simulink model "proje_v1"  (R2016a)
settings: Solver=VariableStepAuto  StartTime=0.0  StopTime=2  RelTol=1e-3
libraries: powerlib x7, electricdrivelib x1
settings Model: Creator=acer  LastModifiedBy=gunge

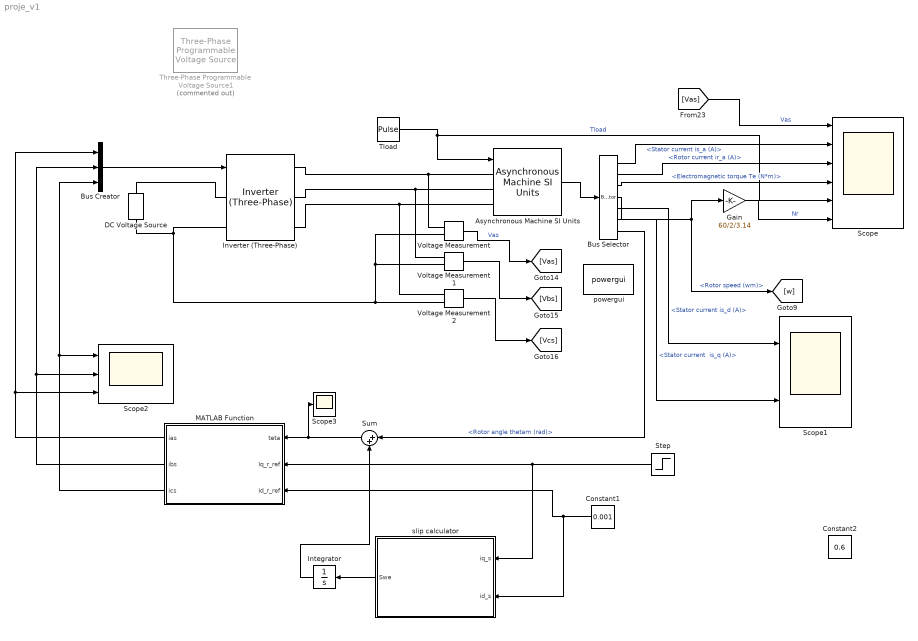
== system proje_v1 ==
  Asynchronous Machine SI Units : powerlib/Machines/Asynchronous Machine SI Units  RotorType=Squirrel-cage  PresetModel=No  MechanicalLoad=Torque Tm  ShowDetailedParameters=on  ReferenceFrame=Rotor  Units=SI  MeasurementBus=off  NominalParameters=[3730 230 60]  Stator=[0.531 0.00252]  Rotor=[0.408 0.00252]  Cage1=[0.4155 0.002066]  Cage2=[0.4168 0.0003495]  Lm=0.0847  Mechanical=[0.1 0 2]  PolePairs=2  InitialConditions=[1 0 0 0 0 0 0 0]  SimulateSaturation=off  Saturation=[14.03593122, 27.81365428, 53.79336849, 72.68890987, 97.98006896, 148.6815601, 215.7428561, 302.9841135, 428.7778367 ; 230, 322, 414, 460, 506, 552, 598, 644, 690]  LoadFlowParameters=1492000  TsPowergui=0  TsBlock=-1  IterativeModel=Trapezoidal non iterative  IterativeDiscreteModel=Trapezoidal non iterative  Pmec=1.492e+006
  Bus Creator : BusCreator  Inputs=3
  Bus Selector : BusSelector  OutputSignals="Stator measurements.Stator current is_a (A),Rotor measurements.Rotor current ir_a (A),Mechanical.Electromagnetic torque Te (N*m),Mechanical.Rotor speed (wm),Stator measurements.Stator current is_d (A),Stator measurements.Stator current  is_q (A),Mechanical.Rotor angle thetam (rad)"
  Constant1 : Constant  Value=0.001
  Constant2 : Constant  Value=0.6
  DC Voltage Source : powerlib/Electrical Sources/DC Voltage Source  Amplitude=540  Measurements=Voltage
  Gain : Gain  Gain=60/2/3.14
  Integrator : Integrator
  Inverter (Three-Phase) : electricdrivelib/Fundamental Drive Blocks/Inverter (Three-Phase)  OverrideUsingVariant=Average_SVM  detailLevel=Average  driveType=Space vector modulation  Ts=2e-6  SnubberResistance=10e3  SnubberCapacitance=inf  Device=IGBT / Diodes  Ron=1e-3  ForwardVoltages=[1.2,1.2]  GTOparameters=[1e-6,2e-6]  IGBTparameters=[1e-6,2e-6]  Measurements=All voltages and currents  converterType=Inverter  SourceFrequency=60  ReferenceFrame=Rotor  dqInductances=[8.5e-3,8.5e-3]  Inductance=8.5e-3  Ls=0  Resistance=0.2  Flux=0.175  Stator_sm=[2.01e-3,4.289e-4,4.477e-3,1.354e-3]  Stator_im=[14.85e-3,0.3027e-3]  Rotor=[9.295e-3,0.3027e-3]  Lm=10.46e-3  p=4
      settings: AttributesFormatString=%<BlockChoice>
  MATLAB Function : MATLAB Function  TreatAsAtomicUnit=on
  Scope : Scope  NumInputPorts=6
  Scope1 : Scope  NumInputPorts=2
  Scope2 : Scope  NumInputPorts=3
  Scope3 : Scope
  Step : Step  Before=0.3  After=0.6  SampleTime=0
  Sum : Sum  Inputs=|++
  Three-Phase Programmable Voltage Source1 : powerlib/Electrical Sources/Three-Phase Programmable Voltage Source  Commented=on  PositiveSequence="[230  0 60]"  VariationEntity=None  VariationType=Table of time-amplitude pairs  VariationTypeAlt=Step  VariationStep=0.5  VariationRate=10  VariationMagnitude=0.3  VariationFrequency=2  VariationTiming=[1 2]  VariationPhaseA=off  Amplitudes=[1 0.8 1.2 1.0]  TimeValues=[0 0.1 0.15 0.2]  HarmonicGeneration=off  HarmonicA=[3 0.2 -25 0]  HarmonicB=[2 0.15 35 2]  Timing="[0.05  3]"  BusType=swing  Pref=0  Qref=0  Qmin=-inf  Qmax=inf
  Tload : DiscretePulseGenerator  PulseType=Time based  Amplitude=15  Period=1  PulseWidth=10  PhaseDelay=0.7
  Voltage Measurement : powerlib/Measurements/Voltage Measurement  PhasorSimulation=off  OutputType=Complex  PSBequivalent=0
  Voltage Measurement1 : powerlib/Measurements/Voltage Measurement  PhasorSimulation=off  OutputType=Complex  PSBequivalent=0
  Voltage Measurement2 : powerlib/Measurements/Voltage Measurement  PhasorSimulation=off  OutputType=Complex  PSBequivalent=0
  powergui : powerlib/powergui  Priority=1  SimulationMode=Discrete  SolverType=Tustin/Backward Euler (TBE)  SampleTime=1e-6  frequency=60  SPID=off  DisableSnubberDevices=off  DisableRonSwitches=off  DisableVfSwitches=off  SwTol=0  DisplayEquations=off  Interpol=off  ExternalGateDelay=off  methode=off  Ts=10  FunctionMessages=off  echomessages=off  HookPort=off  EnableUseOfTLC=off  x0status=blocks  frequencyindice=60  Pbase=100e6  ErrMax=1e-4  Iterations=50  UnitsV=kV  UnitsW=MW  buscounter=0  RestoreLinks=warning  ResistiveCurrentMeasurement=off  Frange=[0:2:500]  Ylog=off  Xlog=on  ShowGrid=off  save=off  variable=ZData  structure=0  ZoomFFT=off  StartTime=0.0  cycles=1  DisplayStyle=1  fundamental=60  FreqAxis=off  MaxFrequency=1000  frequencyindicesteady=1  RmsSteady=1  display=off
  slip calculator : MATLAB Function  TreatAsAtomicUnit=on
  wires:
  Tload/1 -> Scope/5, Asynchronous Machine SI Units/1  "Tload"
  Asynchronous Machine SI Units/1 -> Bus Selector/1
  Bus Selector/1 -> Scope/2  "<Stator current is_a (A)>"
  Bus Selector/2 -> Scope/3  "<Rotor current ir_a (A)>"
  Bus Selector/3 -> Scope/4  "<Electromagnetic torque Te (N*m)>"
  Bus Selector/4 -> Gain/1, [w]  "<Rotor speed (wm)>"
  Gain/1 -> Scope/6  "Nr"
  Voltage Measurement/1 -> [Vas]  "Vas"
  Voltage Measurement1/1 -> [Vbs]
  Voltage Measurement2/1 -> [Vcs]
  [Vas] -> Scope/1  "Vas"
  Bus Selector/5 -> Scope1/1  "<Stator current is_d (A)>"
  Bus Selector/6 -> Scope1/2  "<Stator current  is_q (A)>"
  Bus Creator/1 -> Inverter (Three-Phase)/1
  Bus Selector/7 -> Sum/1  "<Rotor angle thetam (rad)>"
  Step/1 -> slip calculator/1(iq_s), MATLAB Function/2(Iq_r_ref)
  Constant1/1 -> slip calculator/2(id_s), MATLAB Function/3(Id_r_ref)
  MATLAB Function/1(ias) -> Bus Creator/1, Scope2/3
  MATLAB Function/2(ibs) -> Scope2/2, Bus Creator/2
  MATLAB Function/3(ics) -> Bus Creator/3, Scope2/1
  slip calculator/1(Swe) -> Integrator/1
  Integrator/1 -> Sum/2
  Sum/1 -> Scope3/1, MATLAB Function/1(teta)
  connections:
  Voltage Measurement/LConn1 -- Inverter (Three-Phase)/RConn1 -- Asynchronous Machine SI Units/LConn1
  Voltage Measurement1/LConn1 -- Inverter (Three-Phase)/RConn2 -- Asynchronous Machine SI Units/LConn2
  Voltage Measurement2/LConn1 -- Asynchronous Machine SI Units/LConn3 -- Inverter (Three-Phase)/RConn3
  Voltage Measurement/LConn2 -- DC Voltage Source/LConn1 -- Inverter (Three-Phase)/LConn2 -- Voltage Measurement2/LConn2 -- Voltage Measurement1/LConn2
  DC Voltage Source/RConn1 -- Inverter (Three-Phase)/LConn1

== matlab function proje_v1/slip calculator ==
  data: iq_s input; Swe output; id_s input
function Swe = fcn(iq_s,id_s)
%#codegen
Rr = 0.408;
Lr = (2.52+84.7)*10e-3;




Swe = Rr/Lr*iq_s/id_s;

== matlab function proje_v1/MATLAB Function ==
  data: teta input; Iq_r_ref input; ias output; Id_r_ref input; ibs output; ics output
function [ias, ibs ,ics]= fcn(teta,Iq_r_ref,Id_r_ref)
%#codegen


    iq_s = cos(teta)*Iq_r_ref + sin(teta)*Id_r_ref;
    id_s = -sin(teta)*Iq_r_ref + cos(teta)*Id_r_ref;
    
    
ias = iq_s;
ibs =  (-0.5*iq_s - sqrt(3)/2*id_s);
ics = (-ias-ibs);
